simulink model "fan_controller"  (R2019a)
settings: Solver=FixedStepAuto  StartTime=0.0  StopTime=10.0  RelTol=1e-3
libraries: fuzblock x1
settings Model: Creator=edoardo  LastModifiedBy=edoardo
settings OptimizationCC: DefaultParameterBehavior=Inlined  UseDivisionForNetSlopeComputation=on  GainParamInheritBuiltInType=on  UseFloatMulNetSlope=on  InlineInvariantSignals=on  PassReuseOutputArgsAs=Individual arguments  ZeroExternalMemoryAtStartup=off  ZeroInternalMemoryAtStartup=off  NoFixptDivByZeroProtection=on  EfficientFloat2IntCast=on  LifeSpan=1  OptimizeBlockOrder=speed  DifferentSizesBufferReuse=on
settings DebuggingCC: ParameterTunabilityLossMsg=error
settings HardwareCC: ProdBitPerPointer=32  ProdBitPerSizeT=32  ProdBitPerPtrDiffT=32  ProdLargestAtomicInteger=Long  ProdLargestAtomicFloat=Double  ProdWordSize=32  ProdLongLongMode=on  ProdHWDeviceType=ARM Compatible->ARM Cortex
settings SFSimCC: MATLABDynamicMemAlloc=off
settings RTWCC: SystemTargetFile=ert.tlc  TemplateMakefile=ert_default_tmf  GenerateReport=on  IncludeHyperlinkInReport=on  LaunchReport=on  GenerateTraceInfo=on  GenerateTraceReport=on  GenerateTraceReportSl=on  GenerateTraceReportSf=on  GenerateTraceReportEml=on  GenerateCodeMetricsReport=on
settings CodeAppCC: ForceParamTrailComments=on  IgnoreCustomStorageClasses=off  OperatorAnnotations=on  SimulinkDataObjDesc=on  SFDataObjDesc=on  CustomSymbolStrGlobalVar=rt$N$M  CustomSymbolStrType=$N$M  CustomSymbolStrFcn=$N$M$F  CustomSymbolStrMacro=$N$M  InsertBlockDesc=on
settings ERTTargetCC: TargetLangStandard=C99 (ISO)  GenerateSampleERTMain=on  IncludeMdlTerminateFcn=off  CombineSignalStateStructs=on  SupportAbsoluteTime=off  SupportComplex=off  SupportContinuousTime=on  SupportNonInlinedSFcns=on  InlinedParameterPlacement=NonHierarchical  ERTCustomFileTemplate=example_file_process.tlc  ERTFilePackagingFormat=CompactWithDataFile

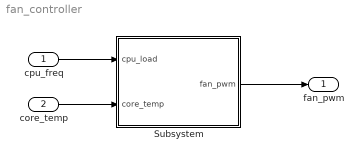
== system fan_controller ==
  cpu_freq : Inport
  core_temp : Inport  Port=2
  Subsystem : Subsystem
  fan_pwm : Outport
  wires:
  cpu_freq/1 -> Subsystem/1(cpu_load)
  core_temp/1 -> Subsystem/2(core_temp)
  Subsystem/1(fan_pwm) -> fan_pwm/1

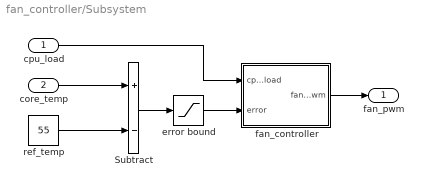
== system fan_controller/Subsystem ==
  cpu_load : Inport
  core_temp : Inport  Port=2
  Subtract : Sum  Inputs=+-
  error bound : Saturate  UpperLimit=80  LowerLimit=0
  "fan_controller " : Subsystem
  ref_temp : Constant  Value=55
  fan_pwm : Outport
  wires:
  ref_temp/1 -> Subtract/2
  cpu_load/1 -> "fan_controller "/1("cpu_load ")
  "fan_controller "/1("fan_pwm ") -> fan_pwm/1
  core_temp/1 -> Subtract/1
  Subtract/1 -> error bound/1
  error bound/1 -> "fan_controller "/2("error ")

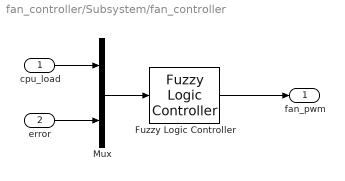
== system fan_controller/Subsystem/fan_controller  ==
  "cpu_load " : Inport
  "error " : Inport  Port=2
  Fuzzy Logic Controller : fuzblock/Fuzzy Logic  Controller  FIS=fan_controller  OutputSampleNumber=101  DataType=double  FuzzifiedInputs=off  RuleFiringStrengths=off  RuleOutputs=off  AggregatedOutputs=off  SimulateUsing=Code generation  OutOfRangeInputValueMessage=error  NoRuleFiredMessage=error  EmptyOutputFuzzySetMessage=error
  Mux : Mux  Inputs=2
  "fan_pwm " : Outport
  wires:
  Fuzzy Logic Controller/1 -> "fan_pwm "/1
  Mux/1 -> Fuzzy Logic Controller/1
  "cpu_load "/1 -> Mux/1
  "error "/1 -> Mux/2
